simulink model "rov_kinematics_level3"  (R2024b)
settings: Solver=ode15s  StartTime=0.0  StopTime=90  FixedStep=0.01  MinStep=1e-6  RelTol=1e-1  AbsTol=1e-3
values from neighbouring files (symbols this model uses):
  A_obs = A_aug - L_sens * C_sens    [main.m]    (also in test_controller_observer.m)
  B_obs = [ B_aug,   L_sens ]    [main.m]    (also in test_controller_observer.m)
  C_int = C(1:ni,:)    [designHoverController.m]    (also in designHoverControllerAtTrim.m = eye(ni,n); main.m = C_aug(1:ni, :); main_hover_controller.m = C_aug(1:ni, :); test_controller_observer.m = [eye(ni), zeros(ni, n-ni)])
  C_obs = eye(n)    [main.m]    (also in test_controller_observer.m)
  D_obs = zeros(n, size(B_obs,2))    [main.m]    (also in test_controller_observer.m)
  F_max = 30    [main.m]    (also in rovWithActuators.m)
  grid_pts = zeros(numel(phi_vals)*numel(theta_vals), 2)    [buildGainGrid.m]
  K = 40    [main.m]    (also in main_hover_controller.m; rovWithActuators.m)
  Ki = Kfull(:, n+1:end)    [designHoverController.m]    (also in designHoverControllerAtTrim.m)
  Ki_all = zeros(m, ni, numel(phi_vals)*numel(theta_vals))    [buildGainGrid.m]
  Kx = Kfull(:, 1:n)    [designHoverController.m]    (also in designHoverControllerAtTrim.m)
  Kx_all = zeros(m, n, numel(phi_vals)*numel(theta_vals))    [buildGainGrid.m]
  tau_act = 0.1    [main.m]
  Tmix = [     [ e1; cross(r1,e1)], [ e2; cross(r2,e2)],      [ e3; cross(r3,e3)], [ e4; cross(r4,e4)],      [ e5; cross(r5,e5)], [ e6; cross(r6,e6)],      [ e7; cross(r7,e7)], [ e8; cross(r8,e8)]     ]    [buildMixingMatrix.m]    (also in main.m = buildMixingMatrix(); main_hover_controller.m = buildMixingMatrix_Xconfig(); rovWithActuators.m = buildMixingMatrix())
libraries: simulink x1
settings Model: Creator=eirikvarnes  LastModifiedBy=eirikvarnes
settings DataIOCC: SaveFormat=Array  SaveTime=off  ReturnWorkspaceOutputs=off  OutputSaveName=eta

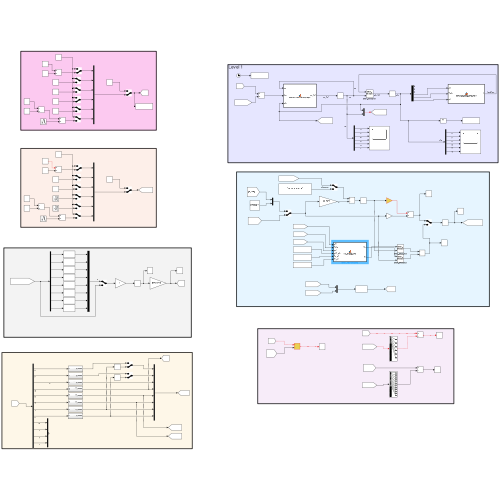
[thumbnail: Simulink's stored preview of the top-level diagram]
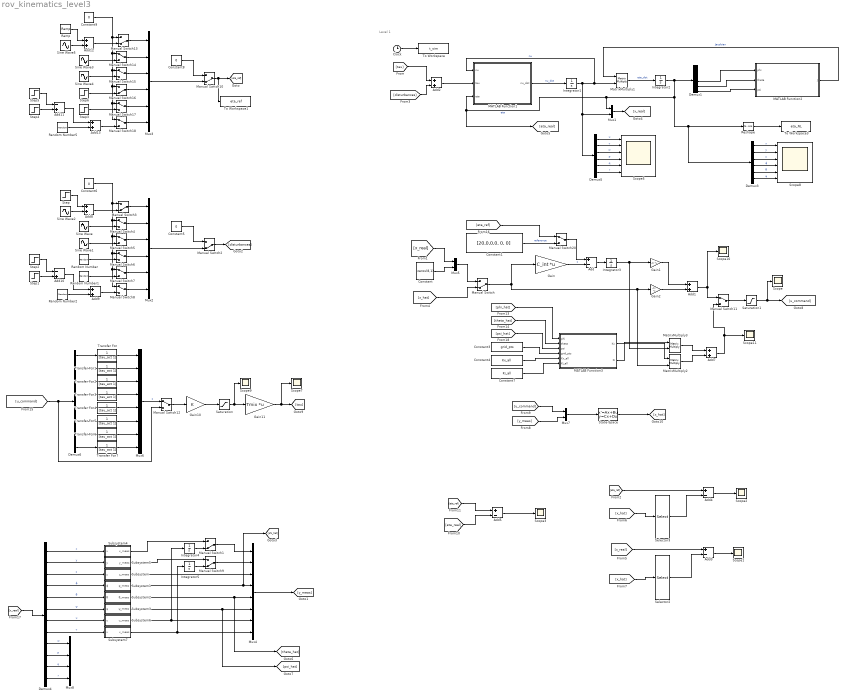
== system rov_kinematics_level3 ==
  note: Level 1
  Add{,3..5} (4 alike) : Sum  Inputs=+-
  Add{1..2,7..9,12..13} (7 alike) : Sum
  Add10 : Sum  Inputs=-+
  Add11 : Sum  Inputs=-+
  Clock : Clock
  Constant : Constant  Value=zeros(8,1)
  Constant1 : Constant  Value=[20,0,0,0, 0, 0]
  Constant3 : Constant  Value=grid_pts
  Constant4 : Constant  Value=Kx_all
  Constant{5..6,8..9} (4 alike) : Constant  Value=0
  Constant7 : Constant  Value=Ki_all
  Demux1 : Demux  Outputs=6
  Demux3 : Demux  Outputs=6
  Demux4 : Demux  Outputs=12
  Demux5 : Demux  Outputs=6
  Demux6 : Demux  Outputs=8
  Gain : Gain  Gain=C_int  Multiplication=Matrix(K*u)
  Gain1 : Gain  Gain=-Ki  Multiplication=Matrix(K*u)
  Gain10 : Gain  Gain=K
  Gain11 : Gain  Gain=Tmix  Multiplication=Matrix(K*u) (u vector)
  Gain2 : Gain  Gain=-Kx  Multiplication=Matrix(K*u)
  Integrator{1..5} (5 alike) : Integrator
  MATLAB Function1 : MATLAB Function  TreatAsAtomicUnit=on
  MATLAB Function2 : MATLAB Function  TreatAsAtomicUnit=on
  MATLAB Function3 : MATLAB Function  TreatAsAtomicUnit=on
  Manual Switch{,1..3,9..10,13,16} (8 alike) : ManualSwitch  CurrentSetting=0
  Manual Switch{4..8,11..12,14..15,17..18,20} (12 alike) : ManualSwitch
  MatrixMultiply1 : Product  Multiplication=Matrix(*)
  MatrixMultiply2 : Product  Multiplication=Matrix(*)
  MatrixMultiply3 : Product  Multiplication=Matrix(*)
  Mux1 : Mux  Inputs=2
  Mux2 : Mux  Inputs=6
  Mux3 : Mux  Inputs=6
  Mux4 : Mux  Inputs=8
  Mux5 : Mux  Inputs=2
  Mux6 : Mux  Inputs=8
  Mux7 : Mux  Inputs=2
  Mux8 : Mux
  Ramp : simulink/Sources/Ramp  slope=1  start=0  InitialOutput=0
  Random Number : RandomNumber  Variance=0.1  SampleTime=0.1
  Random Number1 : RandomNumber  Variance=0.03  SampleTime=0.1
  Random Number2 : RandomNumber  Variance=0.05  SampleTime=0.1
  Random Number5 : RandomNumber  Variance=0.05  SampleTime=0.1
  Reshape : Reshape  OutputDimensionality=Customize  OutputDimensions=[6]
  Saturation : Saturate  UpperLimit=F_max  LowerLimit=-F_max
  Saturation1 : Saturate  UpperLimit=1  LowerLimit=-1
  Scope{,1..3,7,9..11} (8 alike) : Scope
  Scope5 : Scope  NumInputPorts=6
  Scope8 : Scope  NumInputPorts=6
  Selector2 : Selector  InputPortWidth=20  IndexOptions=Index vector (dialog)  Indices=[1 2 3 4 5 6 7 8 9 10 11 12]  OutputSizes=1
  Selector3 : Selector  InputPortWidth=20  IndexOptions=Index vector (dialog)  Indices=[1 2 3 4 5 6]  OutputSizes=1
  Sine Wave : Sin  Amplitude=10  Frequency=0.05  SampleTime=0
  Sine Wave1 : Sin  Amplitude=20  Frequency=0.08  SampleTime=0
  Sine Wave2 : Sin  Amplitude=0.0  Frequency=0.05  SampleTime=0
  Sine Wave3 : Sin  Amplitude=5  Frequency=0.1  SampleTime=0
  Sine Wave4 : Sin  Amplitude=20  Frequency=0.08  SampleTime=0
  Sine Wave5 : Sin  Amplitude=0  Frequency=0.05  SampleTime=0
  State-Space : StateSpace  A=A_obs  B=B_obs  C=C_obs  D=D_obs  InitialCondition=0
  Step : Step  Time=0  After=3  SampleTime=0
  Step1 : Step  Time=5  After=10  SampleTime=2
  Step2 : Step  Time=8  After=10  SampleTime=2
  Step3 : Step  Time=0.0  After=10  SampleTime=2
  Step4 : Step  Time=5  After=10  SampleTime=2
  Step5 : Step  Time=8  After=10  SampleTime=2
  Step6 : Step  Time=0  After=0.5  SampleTime=2
  Subsystem : Subsystem
  Subsystem1 : Subsystem
  Subsystem2 : Subsystem
  Subsystem3 : Subsystem
  Subsystem4 : Subsystem
  Subsystem5 : Subsystem
  Subsystem6 : Subsystem
  Subsystem7 : Subsystem
  To Workspace : ToWorkspace  VariableName=t_sim  SampleTime=-1
  To Workspace1 : ToWorkspace  VariableName=eta_ref  SampleTime=-1
  To Workspace3 : ToWorkspace  VariableName=eta_NL  SampleTime=-1
  Transfer Fcn{,1..7} (8 alike) : TransferFcn  Denominator=[tau_act 1]
  wires:
  MATLAB Function1/1(nu_dot) -> Integrator1/1  "nu_dot"
  MATLAB Function2/1(J) -> MatrixMultiply1/1  "Jacobian"
  Demux1/6 -> MATLAB Function2/3(psi)
  Demux1/4 -> MATLAB Function2/1(phi)
  MatrixMultiply1/1 -> Integrator2/1  "eta_dot"
  Demux1/5 -> MATLAB Function2/2(theta)
  Reshape/1 -> To Workspace3/1
  Constant5/1 -> Manual Switch2/1
  Manual Switch3/1 -> Mux2/1
  Sine Wave/1 -> Manual Switch4/2
  Random Number/1 -> Manual Switch6/2
  Manual Switch7/1 -> Mux2/5
  Manual Switch5/1 -> Mux2/3
  Manual Switch4/1 -> Mux2/2
  Manual Switch6/1 -> Mux2/4
  Mux2/1 -> Manual Switch2/2
  Random Number2/1 -> Add9/2
  Sine Wave2/1 -> Add8/2
  Manual Switch2/1 -> [disturbances]
  Manual Switch8/1 -> Mux2/6
  Constant6/1 -> Manual Switch8/1, Manual Switch7/1, Manual Switch6/1, Manual Switch5/1, Manual Switch4/1, Manual Switch3/1
  Sine Wave1/1 -> Manual Switch5/2
  Random Number1/1 -> Manual Switch7/2
  Add3/1 -> Scope1/1
  [x_real] -> Add3/1
  [x_hat] -> Selector2/1
  Integrator2/1 -> Demux1/1, MATLAB Function1/3(eta), [eta_real], Mux1/1, Demux3/1, Reshape/1  "eta"
  Demux3/1 -> Scope8/1  "x"
  Demux3/5 -> Scope8/5  "θ"
  Demux3/3 -> Scope8/3  "z"
  Demux3/6 -> Scope8/6  "ψ"
  Demux3/4 -> Scope8/4  "ϕ"
  Demux3/2 -> Scope8/2  "y"
  Add2/1 -> MATLAB Function1/2(tau)
  [disturbances] -> Add2/2
  [tau] -> Add2/1
  Demux5/2 -> Scope5/2  "v"
  Demux5/5 -> Scope5/5  "q"
  Demux5/1 -> Scope5/1  "u"
  Demux5/4 -> Scope5/4  "p"
  Demux5/3 -> Scope5/3  "w"
  Demux5/6 -> Scope5/6  "r"
  Integrator1/1 -> Demux5/1, Mux1/2, MATLAB Function1/1(nu), MatrixMultiply1/2  "nu"
  Mux1/1 -> [x_real]
  Clock/1 -> To Workspace/1
  [x_hat] -> Manual Switch/2
  Mux6/1 -> Manual Switch12/1  "z"
  Gain10/1 -> Saturation/1
  Add1/1 -> Scope10/1, Manual Switch11/1
  Saturation/1 -> Scope9/1, Gain11/1
  Demux6/1 -> Transfer Fcn/1
  Transfer Fcn/1 -> Mux6/1
  Demux6/2 -> Transfer Fcn1/1
  Transfer Fcn1/1 -> Mux6/2
  Demux6/3 -> Transfer Fcn2/1
  Transfer Fcn2/1 -> Mux6/3
  Demux6/4 -> Transfer Fcn3/1
  Transfer Fcn3/1 -> Mux6/4
  Demux6/5 -> Transfer Fcn4/1
  Transfer Fcn4/1 -> Mux6/5
  Demux6/6 -> Transfer Fcn5/1
  Transfer Fcn5/1 -> Mux6/6
  Demux6/7 -> Transfer Fcn6/1
  Transfer Fcn6/1 -> Mux6/7
  Demux6/8 -> Transfer Fcn7/1
  Transfer Fcn7/1 -> Mux6/8
  Saturation1/1 -> Scope/1, [u_command]
  [u_command] -> Manual Switch12/2, Demux6/1
  Gain11/1 -> Scope7/1, [tau]
  Gain/1 -> Add/2  "z"
  Add/1 -> Integrator3/1
  Constant1/1 -> Manual Switch20/2  "reference"
  Manual Switch/1 -> MatrixMultiply2/2, Gain2/1, Gain/1
  [u_command] -> Mux7/1
  State-Space/1 -> [x_hat]
  Selector2/1 -> Add3/2
  Add4/1 -> Scope2/1
  [x_hat] -> Selector3/1
  [eta_ref] -> Add4/1
  Selector3/1 -> Add4/2
  Mux5/1 -> Manual Switch/1
  Constant/1 -> Mux5/2
  [x_real] -> Mux5/1
  Demux4/1 -> Subsystem4/1(x)  "x"
  Demux4/4 -> Subsystem1/1(ϕ)  "ϕ"
  Demux4/5 -> Subsystem2/1(θ)  "θ"
  Demux4/2 -> Subsystem5/1(y)  "y"
  Demux4/6 -> Subsystem3/1(ψ)  "ψ"
  Demux4/10 -> Mux8/2  "p"
  Demux4/8 -> Subsystem7/1(v)  "v"
  Demux4/9 -> Mux8/1  "w"
  Demux4/11 -> Mux8/3  "q"
  Demux4/12 -> Mux8/4  "r"
  Demux4/7 -> Subsystem6/1(u)  "u"
  [x_real] -> Demux4/1
  Demux4/3 -> Subsystem/1(z)  "z"
  Integrator4/1 -> Manual Switch1/2
  Subsystem4/1(x_meas) -> Manual Switch1/1
  Integrator5/1 -> Manual Switch9/2
  Subsystem5/1(y_meas) -> Manual Switch9/1
  Subsystem6/1(u_meas) -> Integrator4/1, Mux4/7
  Subsystem7/1(v_meas) -> Mux4/8, Integrator5/1
  Manual Switch1/1 -> Mux4/1
  Manual Switch9/1 -> Mux4/2
  Subsystem/1(z_meas) -> Mux4/3
  Subsystem1/1(φ_meas) -> [phi_hat], Mux4/4
  Subsystem2/1(θ_meas) -> [theta_hat], Mux4/5
  Subsystem3/1(ψ_meas) -> [psi_hat], Mux4/6
  Add5/1 -> Scope3/1
  [eta_ref] -> Add5/1
  Mux4/1 -> [y_meas]
  Integrator3/1 -> MatrixMultiply3/2, Gain1/1
  Manual Switch11/1 -> Saturation1/1
  Add7/1 -> Manual Switch11/2, Scope11/1
  Constant4/1 -> MATLAB Function3/5(Kx_all)
  MATLAB Function3/2(Ki) -> MatrixMultiply3/1
  Constant3/1 -> MATLAB Function3/4(grid_pts)
  Constant7/1 -> MATLAB Function3/6(Ki_all)
  MATLAB Function3/1(Kx) -> MatrixMultiply2/1
  [phi_hat] -> MATLAB Function3/1(phi)
  [theta_hat] -> MATLAB Function3/2(theta)
  Gain1/1 -> Add1/1
  Gain2/1 -> Add1/2
  MatrixMultiply3/1 -> Add7/1
  MatrixMultiply2/1 -> Add7/2
  Manual Switch12/1 -> Gain10/1
  Step/1 -> Add8/1
  Add8/1 -> Manual Switch3/2
  Add9/1 -> Manual Switch8/2
  Step1/1 -> Add10/2
  Step2/1 -> Add10/1
  Add10/1 -> Add9/1
  Mux7/1 -> State-Space/1
  [y_meas] -> Mux7/2
  [psi_hat] -> MATLAB Function3/3(psi)
  Constant8/1 -> Manual Switch10/1
  Manual Switch10/1 -> To Workspace1/1, [eta_ref]
  Manual Switch14/1 -> Mux3/2
  Manual Switch17/1 -> Mux3/5
  Mux3/1 -> Manual Switch10/2
  Sine Wave5/1 -> Add12/2
  Ramp/1 -> Add12/1
  Step6/1 -> Manual Switch16/2
  Constant9/1 -> Manual Switch18/1, Manual Switch17/1, Manual Switch16/1, Manual Switch15/1, Manual Switch14/1, Manual Switch13/1
  Manual Switch15/1 -> Mux3/3
  Step3/1 -> Manual Switch17/2
  Manual Switch16/1 -> Mux3/4
  Sine Wave3/1 -> Manual Switch14/2
  Manual Switch13/1 -> Mux3/1
  Add11/1 -> Add13/1
  Random Number5/1 -> Add13/2
  Step4/1 -> Add11/2
  Manual Switch18/1 -> Mux3/6
  Sine Wave4/1 -> Manual Switch15/2
  Add12/1 -> Manual Switch13/2
  Step5/1 -> Add11/1
  Add13/1 -> Manual Switch18/2
  Manual Switch20/1 -> Add/1
  [eta_ref] -> Manual Switch20/1
  [eta_real] -> Add5/2

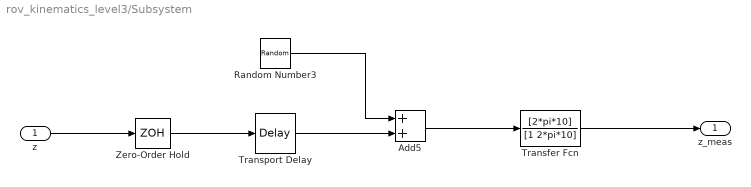
== system rov_kinematics_level3/Subsystem ==
  z : Inport
  Add5 : Sum
  Random Number3 : RandomNumber  Variance=1.5e-5  SampleTime=0.1
  Transfer Fcn : TransferFcn  Numerator=[2*pi*10]  Denominator=[1 2*pi*10]
  Transport Delay : TransportDelay  DelayTime=0
  Zero-Order Hold : ZeroOrderHold  SampleTime=0.05
  z_meas : Outport
  wires:
  z/1 -> Zero-Order Hold/1
  Zero-Order Hold/1 -> Transport Delay/1
  Transport Delay/1 -> Add5/2
  Random Number3/1 -> Add5/1
  Add5/1 -> Transfer Fcn/1
  Transfer Fcn/1 -> z_meas/1

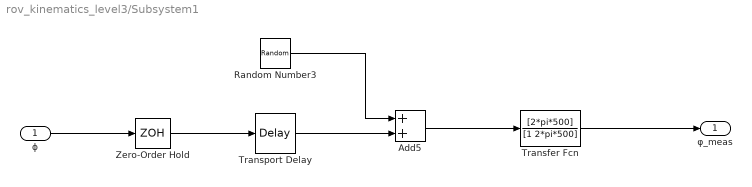
== system rov_kinematics_level3/Subsystem1 ==
  ϕ : Inport
  Add5 : Sum
  Random Number3 : RandomNumber  Variance=2.5e-5  SampleTime=0.1
  Transfer Fcn : TransferFcn  Numerator=[2*pi*500]  Denominator=[1 2*pi*500]
  Transport Delay : TransportDelay  DelayTime=0
  Zero-Order Hold : ZeroOrderHold  SampleTime=0.01
  φ_meas : Outport
  wires:
  ϕ/1 -> Zero-Order Hold/1
  Zero-Order Hold/1 -> Transport Delay/1
  Transport Delay/1 -> Add5/2
  Random Number3/1 -> Add5/1
  Add5/1 -> Transfer Fcn/1
  Transfer Fcn/1 -> φ_meas/1

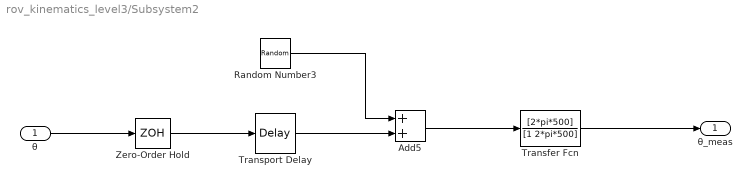
== system rov_kinematics_level3/Subsystem2 ==
  θ : Inport
  Add5 : Sum
  Random Number3 : RandomNumber  Variance=2.5e-5  SampleTime=0.1
  Transfer Fcn : TransferFcn  Numerator=[2*pi*500]  Denominator=[1 2*pi*500]
  Transport Delay : TransportDelay  DelayTime=0
  Zero-Order Hold : ZeroOrderHold  SampleTime=0.01
  θ_meas : Outport
  wires:
  θ/1 -> Zero-Order Hold/1
  Zero-Order Hold/1 -> Transport Delay/1
  Transport Delay/1 -> Add5/2
  Random Number3/1 -> Add5/1
  Add5/1 -> Transfer Fcn/1
  Transfer Fcn/1 -> θ_meas/1

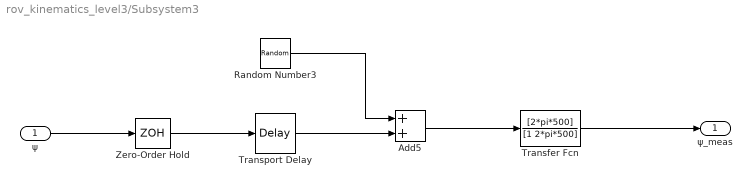
== system rov_kinematics_level3/Subsystem3 ==
  ψ : Inport
  Add5 : Sum
  Random Number3 : RandomNumber  Variance=1.5e-5  SampleTime=0.1
  Transfer Fcn : TransferFcn  Numerator=[2*pi*500]  Denominator=[1 2*pi*500]
  Transport Delay : TransportDelay  DelayTime=0
  Zero-Order Hold : ZeroOrderHold  SampleTime=0.001
  ψ_meas : Outport
  wires:
  ψ/1 -> Zero-Order Hold/1
  Zero-Order Hold/1 -> Transport Delay/1
  Transport Delay/1 -> Add5/2
  Random Number3/1 -> Add5/1
  Add5/1 -> Transfer Fcn/1
  Transfer Fcn/1 -> ψ_meas/1

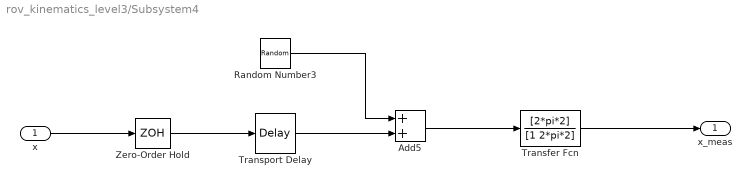
== system rov_kinematics_level3/Subsystem4 ==
  x : Inport
  Add5 : Sum
  Random Number3 : RandomNumber  Variance=1.3e-3  SampleTime=0.1
  Transfer Fcn : TransferFcn  Numerator=[2*pi*2]  Denominator=[1 2*pi*2]
  Transport Delay : TransportDelay  DelayTime=1.2
  Zero-Order Hold : ZeroOrderHold  SampleTime=0.25
  x_meas : Outport
  wires:
  x/1 -> Zero-Order Hold/1
  Zero-Order Hold/1 -> Transport Delay/1
  Transport Delay/1 -> Add5/2
  Random Number3/1 -> Add5/1
  Add5/1 -> Transfer Fcn/1
  Transfer Fcn/1 -> x_meas/1

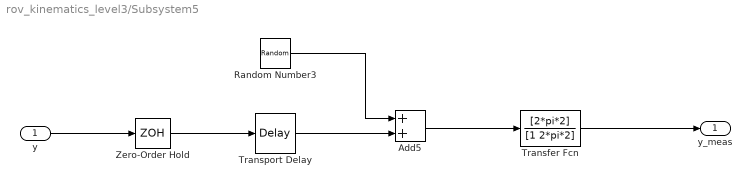
== system rov_kinematics_level3/Subsystem5 ==
  y : Inport
  Add5 : Sum
  Random Number3 : RandomNumber  Variance=1.3e-3  SampleTime=0.1
  Transfer Fcn : TransferFcn  Numerator=[2*pi*2]  Denominator=[1 2*pi*2]
  Transport Delay : TransportDelay  DelayTime=1.2
  Zero-Order Hold : ZeroOrderHold  SampleTime=0.25
  y_meas : Outport
  wires:
  y/1 -> Zero-Order Hold/1
  Zero-Order Hold/1 -> Transport Delay/1
  Transport Delay/1 -> Add5/2
  Random Number3/1 -> Add5/1
  Add5/1 -> Transfer Fcn/1
  Transfer Fcn/1 -> y_meas/1

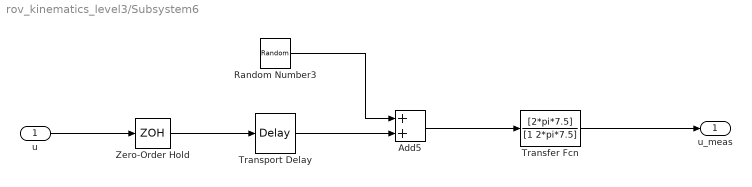
== system rov_kinematics_level3/Subsystem6 ==
  u : Inport
  Add5 : Sum
  Random Number3 : RandomNumber  Variance=0.005  SampleTime=0.1
  Transfer Fcn : TransferFcn  Numerator=[2*pi*7.5]  Denominator=[1 2*pi*7.5]
  Transport Delay : TransportDelay  DelayTime=0.1
  Zero-Order Hold : ZeroOrderHold  SampleTime=0.0667
  u_meas : Outport
  wires:
  u/1 -> Zero-Order Hold/1
  Zero-Order Hold/1 -> Transport Delay/1
  Transport Delay/1 -> Add5/2
  Random Number3/1 -> Add5/1
  Add5/1 -> Transfer Fcn/1
  Transfer Fcn/1 -> u_meas/1

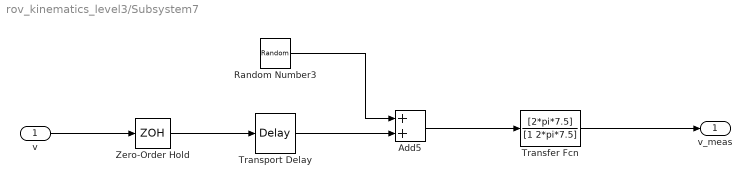
== system rov_kinematics_level3/Subsystem7 ==
  v : Inport
  Add5 : Sum
  Random Number3 : RandomNumber  Variance=0.005  SampleTime=0.1
  Transfer Fcn : TransferFcn  Numerator=[2*pi*7.5]  Denominator=[1 2*pi*7.5]
  Transport Delay : TransportDelay  DelayTime=0.1
  Zero-Order Hold : ZeroOrderHold  SampleTime=0.0667
  v_meas : Outport
  wires:
  v/1 -> Zero-Order Hold/1
  Zero-Order Hold/1 -> Transport Delay/1
  Transport Delay/1 -> Add5/2
  Random Number3/1 -> Add5/1
  Add5/1 -> Transfer Fcn/1
  Transfer Fcn/1 -> v_meas/1

== matlab function rov_kinematics_level3/MATLAB Function1 ==
  data: nu input size=[6 1]; tau input; nu_dot output size=[6 1]; eta input
function nu_dot = computeDynamicsSimple(nu, tau, eta)
% Simplified 6-DOF + small restoring moments for roll/pitch (no heave)
%
% Inputs:
%   nu  [6×1], tau [6×1], eta [6×1]
%
  %#codegen
  p = rovParameters();

  % Rigid‐body inertia
  M_rb = [ p.mass*eye(3), zeros(3);
           zeros(3),       p.I ];

  % Flip vertical thrust
  tau(3) = -tau(3);

  % Drag
  D    = diag(p.D_lin) + diag(p.D_quad .* abs(nu));
  drag = D * nu;

  % Small roll/pitch restoring (no heave)
  phi   = eta(4);
  theta = eta(5);
  K_phi   = p.mass * 0.1;   % small stiffness gains
  K_theta = p.mass * 0.1;
  g = zeros(6,1);
  g(4) = -K_phi   * phi;  
  g(5) = -K_theta * theta;

  % Acceleration
  nu_dot = M_rb \ (tau - drag - g);
end

== matlab function rov_kinematics_level3/MATLAB Function2 ==
  data: phi input; J output; theta input; psi input
function J = computeJacobianSimple(phi, theta, psi)
% ZYX Euler Jacobian, smooth pitch‐singularity clamp

  %#codegen
  cph = cos(phi);   sph = sin(phi);
  cth = cos(theta); sth = sin(theta);
  cps = cos(psi);   sps = sin(psi);

  Rz = [cps,-sps,0; sps,cps,0; 0,0,1];
  Ry = [cth,0,sth; 0,1,0; -sth,0,cth];
  Rx = [1,0,0; 0,cph,-sph; 0,sph,cph];
  R  = Rz * Ry * Rx;

  % smooth clamp
  eps_th = 1e-3;
  safe_ct = sqrt(cth*cth + eps_th*eps_th);

  T = [ ...
    1,  sph*(sth/safe_ct),  cph*(sth/safe_ct);
    0,             cph,              -sph;
    0,      sph/safe_ct,      cph/safe_ct ];

  J = [R, zeros(3); zeros(3), T];
end

== matlab function rov_kinematics_level3/MATLAB Function3 ==
  data: Kx output; Ki output; phi input; theta input; psi input; grid_pts input; Kx_all input; Ki_all input
function [Kx, Ki] = scheduleGains(phi, theta, psi, grid_pts, Kx_all, Ki_all)
  %#codegen
  m = size(Kx_all,1);
  n = size(Kx_all,2);
  Kx = zeros(m,n);
  Ki = zeros(m,6);

  % roll & pitch diffs (linear)
  dphi   = grid_pts(:,1) - phi;
  dtheta = grid_pts(:,2) - theta;

  % yaw diff, wrapped into [-pi,pi]
  dpsi_raw = grid_pts(:,3) - psi;
  dpsi     = atan2(sin(dpsi_raw), cos(dpsi_raw));

  % squared distances
  d2 = dphi.^2 + dtheta.^2 + dpsi.^2;

  % pick nearest
  [~, idx] = min(d2);

  % output gains
  Kx(:,:) = -Kx_all(:,:,idx);
  Ki(:,:) = -Ki_all(:,:,idx);
end
